simulink model "volo_radio_controller"  (Simulink 8.0)
settings: Solver=ode45  SolverMode=SingleTasking  StartTime=0.0  StopTime=1000  RelTol=1e-3
InitFcn:
  | volo_radio_controller_init
values from neighbouring files (symbols this model uses):
  cFI = fi(cMult, 1, 13, 11)    [volo_radio_controller_init.m]
  gFI = fi(gain, 1, 13, 11)    [volo_radio_controller_init.m]
  sFI = fi(sMult, 1, 13, 11)    [volo_radio_controller_init.m]
undefined symbols (not defined in the file or in its folder): gcbh, xlBlockLoadCallback, xlGetNormalizedPeriod, xlipgetpartsetting
libraries: xbsIndex_r4 x380, xbsEDKLib_r4 x1
(part 3 of 5)

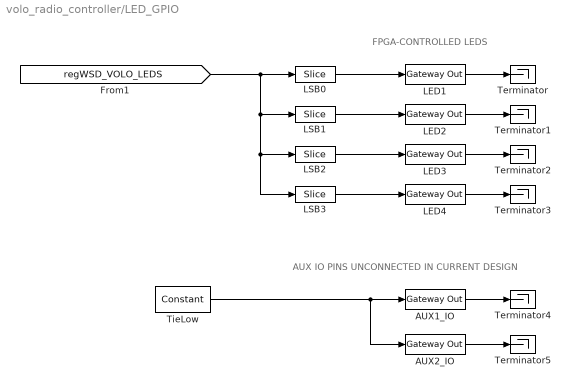
== system volo_radio_controller/LED_GPIO ==
  note: FPGA-CONTROLLED LEDS
  note: AUX IO PINS UNCONNECTED IN CURRENT DESIGN
  AUX1_IO : xbsIndex_r4/Gateway Out  inherit_from_input=off  hdl_port=off  timing_constraint=None  locs_specified=off  LOCs={}  UseAsDAC=off  DACChannel='1'  block_type=gatewayout
      settings: xl_area=[0 0 0 0 1 0 0]
  AUX2_IO : xbsIndex_r4/Gateway Out  inherit_from_input=off  hdl_port=off  timing_constraint=None  locs_specified=off  LOCs={}  UseAsDAC=off  DACChannel='1'  block_type=gatewayout
      settings: xl_area=[0 0 0 0 1 0 0]
  LED{1..4} (4 alike) : xbsIndex_r4/Gateway Out  inherit_from_input=off  hdl_port=on  timing_constraint=None  locs_specified=off  LOCs={}  UseAsDAC=off  DACChannel='1'  block_type=gatewayout
      settings: infoedit="Gateway out block.  Converts Xilinx fixed-point or floating-point type inputs into ouputs of type Simulink integer, single, double, or fixed point.<br><br>Hardware notes:  In hardware these blocks become top level output ports or are discarded, depending on how they are configured."  xl_area=[0 0 0 0 1 0 0]
  LSB0 : xbsIndex_r4/Slice  nbits=1  boolean_output=off  mode=Lower Bit Location + Width  bit1=0  base1=MSB of Input  bit0=0  base0=LSB of Input  dbl_ovrd=off  block_type=slice
      settings: block_version=8.2
  LSB1 : xbsIndex_r4/Slice  nbits=1  boolean_output=off  mode=Lower Bit Location + Width  bit1=0  base1=MSB of Input  bit0=1  base0=LSB of Input  dbl_ovrd=off  block_type=slice
      settings: block_version=8.2
  LSB2 : xbsIndex_r4/Slice  nbits=1  boolean_output=off  mode=Lower Bit Location + Width  bit1=0  base1=MSB of Input  bit0=2  base0=LSB of Input  dbl_ovrd=off  block_type=slice
      settings: block_version=8.2
  LSB3 : xbsIndex_r4/Slice  nbits=1  boolean_output=off  mode=Lower Bit Location + Width  bit1=0  base1=MSB of Input  bit0=3  base0=LSB of Input  dbl_ovrd=off  block_type=slice
      settings: block_version=8.2
  Terminator{,1..5} (6 alike) : Terminator
  TieLow : xbsIndex_r4/Constant  const=0  gui_display_data_type=Fixed-point  arith_type=Unsigned  n_bits=1  bin_pt=0  preci_type=Single  exp_width=8  frac_width=24  explicit_period=off  period=1  equ=P=C  opselect=C  inp2=PCIN>>17  opr=+  inp1=P  carry=CIN  dbl_ovrd=off  block_type=constant
  wires:
  LED1/1 -> Terminator/1
  LED2/1 -> Terminator1/1
  LED3/1 -> Terminator2/1
  LED4/1 -> Terminator3/1
  AUX1_IO/1 -> Terminator4/1
  AUX2_IO/1 -> Terminator5/1
  LSB0/1 -> LED1/1
  LSB1/1 -> LED2/1
  LSB2/1 -> LED3/1
  LSB3/1 -> LED4/1
  [regWSD_VOLO_LEDS] -> LSB0/1, LSB1/1, LSB2/1, LSB3/1
  TieLow/1 -> AUX1_IO/1, AUX2_IO/1

== system volo_radio_controller/Older Revision Notes ==
  note: Ryan - August 05, 2013
      | -------------------------------------
      | Naren - August 13, 2013 - 4.00.d
      | ** Added FP multiplies to IQ Calibration **
      | -----------------------------------
      | Ryan - August 21, 2013 - 4.00.e
      | Replaced Tx/Rx switching delay with single
      | one-shot rather than multiple delay lines:
      | regWSD_TxRxSwitchingDelayCount
      | -----------------------------------
      | 4.00.f - August 24 - Added internal UART out lines
      | with a sane naming convention such that it's easy:
      | internat TX to internal TX, external TX to external TX REG
      | -----------------------------------
      | 4.00.g - Sept 25, 2013 - Modified TXMUX to replace match-filtered
      | Rx loopback with constant-zero signals. This should help
      | with automatic calibration. REG
      | -----------------------------------
      | 4.00.h - Oct 1, 2013 - Added "ISSWAPPED" option to DDS in order
      | to programmatically mirror the SSB exponential across DC. This lets
      | us match the calibration proceedure Lime provided exactly. REG.
      | -----------------------------------
      | 4.00.j - Oct 2, 2013 - Added "ALIGNTESTACTIVE" option to DDS so
      | we can test the I/Q phase alignment. This is a test mode ONLY. REG.
      | -----------------------------------
      | 4.00.k - Oct 13, 2013 - Added "WSD_RXSWITCHINGDELAYCOUNT",
      | "WSD_SPIWAITDELAYCOUNT," and "regWSD_En_ForceSPILow" registers
      | and enable bits in order to control new Tx/Rx delay blocks in the radio controller.
      | The idea behind these is to provide the switching delays required by the SPI,
      | but in a configurable manner. Also delegate between AGC and Tx/Rx swtiching control
      | of the LMS SPI bus. This will be tricky.
      | -----------------------------------

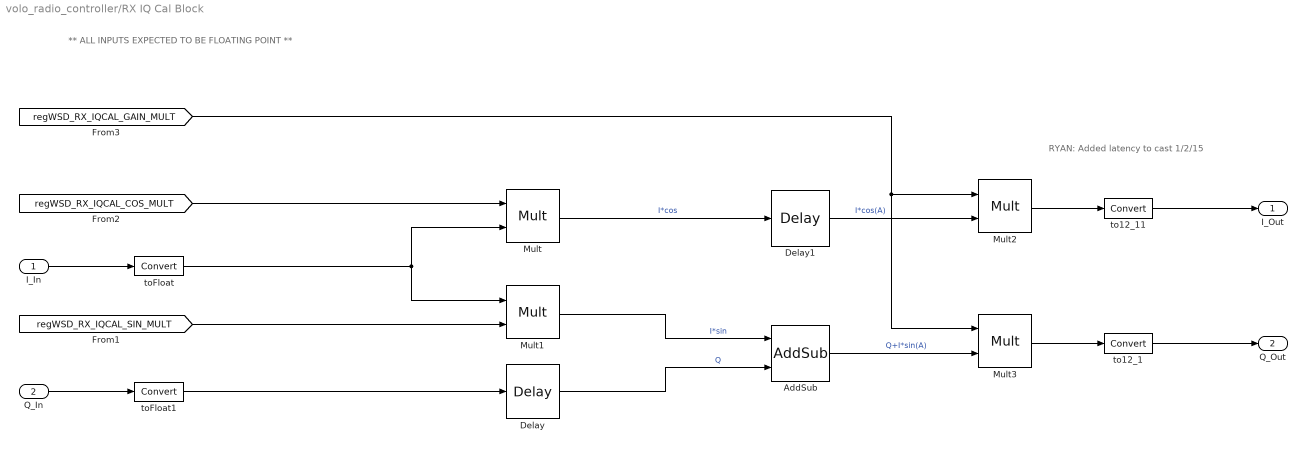
== system volo_radio_controller/RX IQ Cal Block ==
  note: RYAN: Added latency to cast 1/2/15
  note: ** ALL INPUTS EXPECTED TO BE FLOATING POINT **
  I_In : Inport
  Q_In : Inport  Port=2
  AddSub : xbsIndex_r4/AddSub  mode=Addition  use_carryin=off  use_carryout=off  en=off  latency=1  precision=Full  arith_type="Signed  (2's comp)"  n_bits=13  bin_pt=11  quantization="Round  (unbiased: +/- Inf)"  overflow=Flag as error  dbl_ovrd=off  use_behavioral_HDL=off  hw_selection=Fabric  pipelined=off  block_type=addsub
  Delay : xbsIndex_r4/Delay  rst=off  infoeditControl=Selection of Reset will increase slice count due to use of real FFs and instead of SRLs  en=off  latency=3  dbl_ovrd=off  reg_retiming=off  block_type=delay
  Delay1 : xbsIndex_r4/Delay  rst=off  infoeditControl=Selection of Reset will increase slice count due to use of real FFs and instead of SRLs  en=off  latency=1  dbl_ovrd=off  reg_retiming=off  block_type=delay
  Mult : xbsIndex_r4/Mult  precision=Full  arith_type="Signed  (2's comp)"  n_bits=13  bin_pt=11  quantization="Round  (unbiased: +/- Inf)"  overflow=Saturate  en=off  latency=3  dbl_ovrd=off  use_behavioral_HDL=off  opt=Speed  use_embedded=on  optimum_pipeline=off  pipeline=on  use_rpm=on  placement_style=Triangular  block_type=mult
  Mult1 : xbsIndex_r4/Mult  precision=Full  arith_type="Signed  (2's comp)"  n_bits=13  bin_pt=11  quantization="Round  (unbiased: +/- Inf)"  overflow=Saturate  en=off  latency=3  dbl_ovrd=off  use_behavioral_HDL=off  opt=Speed  use_embedded=on  optimum_pipeline=off  pipeline=on  use_rpm=on  placement_style=Triangular  block_type=mult
  Mult2 : xbsIndex_r4/Mult  precision=Full  arith_type="Signed  (2's comp)"  n_bits=12  bin_pt=11  quantization="Round  (unbiased: +/- Inf)"  overflow=Flag as error  en=off  latency=3  dbl_ovrd=off  use_behavioral_HDL=off  opt=Speed  use_embedded=on  optimum_pipeline=off  pipeline=on  use_rpm=on  placement_style=Triangular  block_type=mult
  Mult3 : xbsIndex_r4/Mult  precision=Full  arith_type="Signed  (2's comp)"  n_bits=12  bin_pt=11  quantization="Round  (unbiased: +/- Inf)"  overflow=Saturate  en=off  latency=3  dbl_ovrd=off  use_behavioral_HDL=off  opt=Speed  use_embedded=on  optimum_pipeline=off  pipeline=on  use_rpm=on  placement_style=Triangular  block_type=mult
  to12_1 : xbsIndex_r4/Convert  gui_display_data_type=Fixed-point  arith_type="Signed  (2's comp)"  n_bits=12  bin_pt=11  float_type=Single  exp_bits=8  fraction_bits=24  quantization="Round  (unbiased: +/- Inf)"  overflow=Saturate  en=off  latency=1  dbl_ovrd=off  pipeline=off  block_type=convert
  to12_11 : xbsIndex_r4/Convert  gui_display_data_type=Fixed-point  arith_type="Signed  (2's comp)"  n_bits=12  bin_pt=11  float_type=Single  exp_bits=8  fraction_bits=24  quantization="Round  (unbiased: +/- Inf)"  overflow=Saturate  en=off  latency=1  dbl_ovrd=off  pipeline=off  block_type=convert
  toFloat : xbsIndex_r4/Convert  gui_display_data_type=Floating-point  arith_type=Floating-point  n_bits=13  bin_pt=11  float_type=Single  exp_bits=8  fraction_bits=24  quantization="Round  (unbiased: +/- Inf)"  overflow=Flag as error  en=off  latency=0  dbl_ovrd=off  pipeline=off  block_type=convert
  toFloat1 : xbsIndex_r4/Convert  gui_display_data_type=Floating-point  arith_type=Floating-point  n_bits=13  bin_pt=11  float_type=Single  exp_bits=8  fraction_bits=24  quantization="Round  (unbiased: +/- Inf)"  overflow=Flag as error  en=off  latency=0  dbl_ovrd=off  pipeline=off  block_type=convert
  I_Out : Outport
  Q_Out : Outport  Port=2
  wires:
  I_In/1 -> toFloat/1
  [regWSD_RX_IQCAL_COS_MULT] -> Mult/1
  Q_In/1 -> toFloat1/1
  Mult/1 -> Delay1/1  "I*cos"
  Mult1/1 -> AddSub/1  "I*sin"
  [regWSD_RX_IQCAL_GAIN_MULT] -> Mult3/1, Mult2/1
  Mult2/1 -> to12_11/1
  Mult3/1 -> to12_1/1
  Delay1/1 -> Mult2/2  "I*cos(A)"
  AddSub/1 -> Mult3/2  "Q+I*sin(A)"
  Delay/1 -> AddSub/2  "Q"
  [regWSD_RX_IQCAL_SIN_MULT] -> Mult1/2
  toFloat/1 -> Mult/2, Mult1/1
  toFloat1/1 -> Delay/1
  to12_11/1 -> I_Out/1
  to12_1/1 -> Q_Out/1

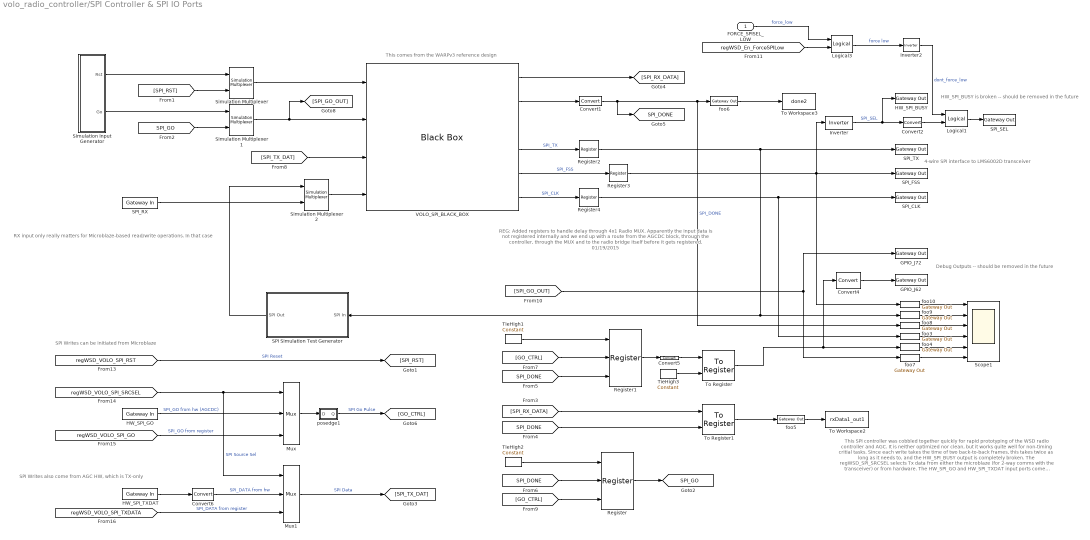
== system volo_radio_controller/SPI Controller & SPI IO Ports ==
  note: REG: Added registers to handle delay through 4x1 Radio MUX.
      | Apparently the input data is not registered internally and we end
      | up with a route from the AGCDC block, through the controller,
      | through the MUX and to the radio bridge itself before it gets
      | registered. 01/19/2015
  note: This comes from the WARPv3 reference design
  note: RX input only really matters for Microblaze-based
      | read/write operations. In that case
  note: This SPI controller was cobbled together quickly
      | for rapid prototyping of the WSD radio controller
      | and AGC. It is neither optimized nor clean, but it
      | works quite well for non-timing critial tasks. Since
      | each write takes the time of two back-to-back
      | frames, this takes twice as long as it needs to, and
      | the HW_SPI_BUSY output is completely broken.
      |
      | The regWSD_SPI_SRCSEL selects Tx data from
      | either the microblaze (for 2-way comms with the
      | transceiver) or from hardware. The HW_SPI_GO
      | and HW_SPI_TXDAT input ports come directly
      | from the WSD_AGCDC block
      |
      | Created: June 2013
      | Author: Narendra Anand (nanand@rice.edu)
      | Comments: Ryan E. Guerra (me@ryaneguerra.com)
  note: SPI Writes also come
      | from AGC HW, which is TX-only
  note: SPI Writes can be initiated from Microblaze
  note: 4-wire SPI interface to
      | LMS6002D transceiver
  note: HW_SPI_BUSY is broken -- should be removed in the future
  note: Debug Outputs -- should be removed in the future
  FORCE_SPISEL_LOW : Inport
  Convert1 : xbsIndex_r4/Convert  gui_display_data_type=Boolean  arith_type=Boolean  n_bits=32  bin_pt=0  float_type=Single  exp_bits=8  fraction_bits=24  quantization=Truncate  overflow=Wrap  en=off  latency=0  dbl_ovrd=off  pipeline=off  block_type=convert
  Convert2 : xbsIndex_r4/Convert  gui_display_data_type=Boolean  arith_type=Boolean  n_bits=32  bin_pt=0  float_type=Single  exp_bits=8  fraction_bits=24  quantization=Truncate  overflow=Wrap  en=off  latency=0  dbl_ovrd=off  pipeline=off  block_type=convert
  Convert4 : xbsIndex_r4/Convert  gui_display_data_type=Boolean  arith_type=Boolean  n_bits=32  bin_pt=0  float_type=Single  exp_bits=8  fraction_bits=24  quantization=Truncate  overflow=Wrap  en=off  latency=0  dbl_ovrd=off  pipeline=off  block_type=convert
  Convert5 : xbsIndex_r4/Convert  gui_display_data_type=Fixed-point  arith_type=Unsigned  n_bits=1  bin_pt=0  float_type=Single  exp_bits=8  fraction_bits=24  quantization=Truncate  overflow=Wrap  en=off  latency=0  dbl_ovrd=off  pipeline=off  block_type=convert
  Convert6 : xbsIndex_r4/Convert  gui_display_data_type=Fixed-point  arith_type=Unsigned  n_bits=32  bin_pt=0  float_type=Single  exp_bits=8  fraction_bits=24  quantization=Truncate  overflow=Saturate  en=off  latency=0  dbl_ovrd=off  pipeline=off  block_type=convert
  GPIO_J62 : xbsIndex_r4/Gateway Out  inherit_from_input=off  hdl_port=off  timing_constraint=None  locs_specified=off  LOCs={}  UseAsDAC=off  DACChannel='1'  block_type=gatewayout
      settings: xl_area=[0 0 0 0 1 0 0]
  GPIO_J72 : xbsIndex_r4/Gateway Out  inherit_from_input=off  hdl_port=off  timing_constraint=None  locs_specified=off  LOCs={}  UseAsDAC=off  DACChannel='1'  block_type=gatewayout
      settings: xl_area=[0 0 0 0 1 0 0]
  HW_SPI_BUSY : xbsIndex_r4/Gateway Out  inherit_from_input=off  hdl_port=off  timing_constraint=None  locs_specified=off  LOCs={}  UseAsDAC=off  DACChannel='1'  block_type=gatewayout
      settings: xl_area=[0 0 0 0 1 0 0]
  HW_SPI_GO : xbsIndex_r4/Gateway In  gui_display_data_type=Boolean  arith_type=Boolean  n_bits=1  bin_pt=0  preci_type=Single  exp_width=8  frac_width=24  quantization=Truncate  overflow=Saturate  period=1  dbl_ovrd=off  timing_constraint=None  locs_specified=off  LOCs={}  UseAsADC=off  ADCChannel='1'  inherit_from_input=off  hdl_port=on  block_type=gatewayin
      settings: xl_area=[0 0 0 0 1 0 0]
  HW_SPI_TXDAT : xbsIndex_r4/Gateway In  gui_display_data_type=Fixed-point  arith_type=Unsigned  n_bits=16  bin_pt=0  preci_type=Single  exp_width=8  frac_width=24  quantization=Truncate  overflow=Saturate  period=1  dbl_ovrd=off  timing_constraint=None  locs_specified=off  LOCs={}  UseAsADC=off  ADCChannel='1'  inherit_from_input=off  hdl_port=on  block_type=gatewayin
      settings: xl_area=[0 0 0 0 1 0 0]
  Inverter : xbsIndex_r4/Inverter  en=off  latency=0  dbl_ovrd=off  block_type=inv
  Inverter2 : xbsIndex_r4/Inverter  en=off  latency=0  dbl_ovrd=off  block_type=inv
  Logical1 : xbsIndex_r4/Logical  logical_function=AND  inputs=2  en=off  latency=0  precision=Full  arith_type=Unsigned  n_bits=16  bin_pt=0  align_bp=on  dbl_ovrd=off  block_type=logical
  Logical3 : xbsIndex_r4/Logical  logical_function=AND  inputs=2  en=off  latency=0  precision=Full  arith_type=Unsigned  n_bits=16  bin_pt=0  align_bp=on  dbl_ovrd=off  block_type=logical
  Mux : xbsIndex_r4/Mux  inputs=2  en=off  latency=0  precision=Full  arith_type=Unsigned  n_bits=16  bin_pt=14  quantization=Truncate  overflow=Wrap  dbl_ovrd=off  block_type=mux
  Mux1 : xbsIndex_r4/Mux  inputs=2  en=off  latency=0  precision=Full  arith_type=Unsigned  n_bits=16  bin_pt=14  quantization=Truncate  overflow=Wrap  dbl_ovrd=off  block_type=mux
  Register : xbsIndex_r4/Register  init=0  rst=on  en=on  dbl_ovrd=off  block_type=register
  Register1 : xbsIndex_r4/Register  init=0  rst=on  en=on  dbl_ovrd=off  block_type=register
  Register2 : xbsIndex_r4/Register  init=0  rst=off  en=off  dbl_ovrd=off  block_type=register
  Register3 : xbsIndex_r4/Register  init=0  rst=off  en=off  dbl_ovrd=off  block_type=register
  Register4 : xbsIndex_r4/Register  init=0  rst=off  en=off  dbl_ovrd=off  block_type=register
  SPI Simulation Test Generator : Subsystem
  SPI_CLK : xbsIndex_r4/Gateway Out  inherit_from_input=off  hdl_port=on  timing_constraint=None  locs_specified=off  LOCs={}  UseAsDAC=off  DACChannel='1'  block_type=gatewayout
      settings: infoedit="Gateway out block.  Converts Xilinx fixed-point or floating-point type inputs into ouputs of type Simulink integer, single, double, or fixed point.<br><br>Hardware notes:  In hardware these blocks become top level output ports or are discarded, depending on how they are configured."  xl_area=[0 0 0 0 1 0 0]
  SPI_FSS : xbsIndex_r4/Gateway Out  inherit_from_input=off  hdl_port=on  timing_constraint=None  locs_specified=off  LOCs={}  UseAsDAC=off  DACChannel='1'  block_type=gatewayout
      settings: infoedit="Gateway out block.  Converts Xilinx fixed-point or floating-point type inputs into ouputs of type Simulink integer, single, double, or fixed point.<br><br>Hardware notes:  In hardware these blocks become top level output ports or are discarded, depending on how they are configured."  xl_area=[0 0 0 0 1 0 0]
  SPI_RX : xbsIndex_r4/Gateway In  gui_display_data_type=Fixed-point  arith_type=Unsigned  n_bits=1  bin_pt=0  preci_type=Single  exp_width=8  frac_width=24  quantization=Truncate  overflow=Saturate  period=1  dbl_ovrd=off  timing_constraint=None  locs_specified=off  LOCs={}  UseAsADC=off  ADCChannel='1'  inherit_from_input=off  hdl_port=on  block_type=gatewayin
      settings: xl_area=[0 0 0 0 1 0 0]
  SPI_SEL : xbsIndex_r4/Gateway Out  inherit_from_input=off  hdl_port=on  timing_constraint=None  locs_specified=off  LOCs={}  UseAsDAC=off  DACChannel='1'  block_type=gatewayout
      settings: infoedit="Gateway out block.  Converts Xilinx fixed-point or floating-point type inputs into ouputs of type Simulink integer, single, double, or fixed point.<br><br>Hardware notes:  In hardware these blocks become top level output ports or are discarded, depending on how they are configured."  xl_area=[0 0 0 0 1 0 0]
  SPI_TX : xbsIndex_r4/Gateway Out  inherit_from_input=off  hdl_port=on  timing_constraint=None  locs_specified=off  LOCs={}  UseAsDAC=off  DACChannel='1'  block_type=gatewayout
      settings: infoedit="Gateway out block.  Converts Xilinx fixed-point or floating-point type inputs into ouputs of type Simulink integer, single, double, or fixed point.<br><br>Hardware notes:  In hardware these blocks become top level output ports or are discarded, depending on how they are configured."  xl_area=[0 0 0 0 1 0 0]
  Scope1 : Scope  NumInputPorts=6
      settings: YMin=-5~-2~-5~-5~-5~-5  YMax=5~2~5~5~5~5
  Simulation Input Generator : Subsystem
  Simulation Multiplexer : xbsIndex_r4/Simulation Multiplexer  sim_sel=1  hw_sel=2  block_type=simmux
      settings: infoedit="Distinguish input subsystems as \"simulation only\" and \"generation only\".  The input specified For Simulation will be used during Simulink simulation.  The input specified For Generation will be used during code generation.  This block will typically be used on the output of a HW Co-Simulation, Black Box, or ModelSim subsystem.<br><br>Hardware Notes: This block costs nothing."
  Simulation Multiplexer1 : xbsIndex_r4/Simulation Multiplexer  sim_sel=1  hw_sel=2  block_type=simmux
      settings: infoedit="Distinguish input subsystems as \"simulation only\" and \"generation only\".  The input specified For Simulation will be used during Simulink simulation.  The input specified For Generation will be used during code generation.  This block will typically be used on the output of a HW Co-Simulation, Black Box, or ModelSim subsystem.<br><br>Hardware Notes: This block costs nothing."
  Simulation Multiplexer2 : xbsIndex_r4/Simulation Multiplexer  sim_sel=1  hw_sel=2  block_type=simmux
      settings: infoedit="Distinguish input subsystems as \"simulation only\" and \"generation only\".  The input specified For Simulation will be used during Simulink simulation.  The input specified For Generation will be used during code generation.  This block will typically be used on the output of a HW Co-Simulation, Black Box, or ModelSim subsystem.<br><br>Hardware Notes: This block costs nothing."
  TieHigh1 : xbsIndex_r4/Constant  const=1  gui_display_data_type=Boolean  arith_type=Boolean  n_bits=1  bin_pt=0  preci_type=Single  exp_width=8  frac_width=24  explicit_period=on  period=1  equ=P=C  opselect=C  inp2=PCIN>>17  opr=+  inp1=P  carry=CIN  dbl_ovrd=off  block_type=constant
  TieHigh2 : xbsIndex_r4/Constant  const=1  gui_display_data_type=Boolean  arith_type=Boolean  n_bits=1  bin_pt=0  preci_type=Single  exp_width=8  frac_width=24  explicit_period=on  period=1  equ=P=C  opselect=C  inp2=PCIN>>17  opr=+  inp1=P  carry=CIN  dbl_ovrd=off  block_type=constant
  TieHigh3 : xbsIndex_r4/Constant  const=1  gui_display_data_type=Boolean  arith_type=Boolean  n_bits=1  bin_pt=0  preci_type=Single  exp_width=8  frac_width=24  explicit_period=on  period=1  equ=P=C  opselect=C  inp2=PCIN>>17  opr=+  inp1=P  carry=CIN  dbl_ovrd=off  block_type=constant
  To Register : xbsIndex_r4/To Register  shared_memory_name='VOLO_SPI_DONE'  init=1  ownership=Locally owned and initialized  explicit_data_type=on  gui_display_data_type=Fixed-point  arith_type=Unsigned  n_bits=1  bin_pt=0  preci_type=Single  dbl_ovrd=off  block_type=toreg
      settings: AttributesFormatString=<< %<shared_memory_name> >>  infoedit="Register block that writes data to a shared memory register.  Delay of one sample period."
  To Register1 : xbsIndex_r4/To Register  shared_memory_name='VOLO_SPI_RXDAT'  init=0  ownership=Locally owned and initialized  explicit_data_type=on  gui_display_data_type=Fixed-point  arith_type=Unsigned  n_bits=32  bin_pt=0  preci_type=Single  dbl_ovrd=off  block_type=toreg
      settings: AttributesFormatString=<< %<shared_memory_name> >>  infoedit="Register block that writes data to a shared memory register.  Delay of one sample period."
  To Workspace2 : ToWorkspace  VariableName=rxData1_out1  SampleTime=-1
  To Workspace3 : ToWorkspace  VariableName=done2  SampleTime=-1
  VOLO_SPI_BLACK_BOX : xbsIndex_r4/Black Box  init_code=volo_spi_io_config  sim_method=ISE Simulator  verbose=off  block_type=blackbox2
  foo{3..10} (8 alike) : xbsIndex_r4/Gateway Out  inherit_from_input=off  hdl_port=off  timing_constraint=None  locs_specified=off  LOCs={}  UseAsDAC=off  DACChannel='1'  block_type=gatewayout
      settings: xl_area=[0 0 0 0 1 0 0]
  posedge1 : Subsystem
  tag scope: SPI_DONE=global, SPI_GO=global
  wires:
  VOLO_SPI_BLACK_BOX/6 -> Register4/1  "SPI_CLK"
  VOLO_SPI_BLACK_BOX/2 -> Convert1/1
  VOLO_SPI_BLACK_BOX/1 -> [SPI_RX_DATA]
  SPI Simulation Test Generator/1(SPI Out) -> Simulation Multiplexer2/1
  Simulation Input Generator/1(Rst) -> Simulation Multiplexer/1
  Simulation Input Generator/2(Go) -> Simulation Multiplexer1/1
  To Register/1 -> Convert4/1, foo4/1
  [SPI_RST] -> Simulation Multiplexer/2
  Simulation Multiplexer/1 -> VOLO_SPI_BLACK_BOX/1
  [regWSD_VOLO_SPI_RST] -> [SPI_RST]  "SPI Reset"
  Convert1/1 -> [SPI_DONE], foo8/1, foo6/1  "SPI_DONE"
  Convert4/1 -> GPIO_J62/1
  [SPI_GO] -> Simulation Multiplexer1/2
  Simulation Multiplexer1/1 -> [SPI_GO_OUT], VOLO_SPI_BLACK_BOX/2
  foo4/1 -> Scope1/5
  foo6/1 -> To Workspace3/1
  VOLO_SPI_BLACK_BOX/4 -> Register2/1  "SPI_TX"
  SPI_RX/1 -> Simulation Multiplexer2/2
  [SPI_TX_DAT] -> VOLO_SPI_BLACK_BOX/3
  Simulation Multiplexer2/1 -> VOLO_SPI_BLACK_BOX/4
  TieHigh2/1 -> Register/1
  Register/1 -> [SPI_GO]
  [SPI_DONE] -> Register/2
  TieHigh3/1 -> To Register/2
  Register1/1 -> Convert5/1
  TieHigh1/1 -> Register1/1
  [SPI_DONE] -> Register1/3
  Convert5/1 -> To Register/1
  [GO_CTRL] -> Register1/2
  posedge1/1(Q) -> [GO_CTRL]  "SPI Go Pulse"
  [GO_CTRL] -> Register/3
  [SPI_GO_OUT] -> GPIO_J72/1, foo7/1
  [regWSD_VOLO_SPI_GO] -> Mux/3  "SPI_GO from register"
  Mux/1 -> posedge1/1(D)
  [regWSD_VOLO_SPI_TXDATA] -> Mux1/3  "SPI_DATA from register"
  Mux1/1 -> [SPI_TX_DAT]  "SPI Data"
  HW_SPI_TXDAT/1 -> Convert6/1
  Convert6/1 -> Mux1/2  "SPI_DATA from hw"
  [regWSD_VOLO_SPI_SRCSEL] -> Mux/1, Mux1/1  "SPI Source Sel"
  Inverter/1 -> HW_SPI_BUSY/1, Convert2/1  "SPI_SEL"
  VOLO_SPI_BLACK_BOX/5 -> Register3/1  "SPI_FSS"
  foo3/1 -> Scope1/4
  [SPI_RX_DATA] -> To Register1/1
  [SPI_DONE] -> To Register1/2
  foo5/1 -> To Workspace2/1
  To Register1/1 -> foo5/1
  foo7/1 -> Scope1/6
  foo8/1 -> Scope1/3
  foo9/1 -> Scope1/2
  foo10/1 -> Scope1/1
  HW_SPI_GO/1 -> Mux/2  "SPI_GO from hw (AGCDC)"
  Logical1/1 -> SPI_SEL/1
  FORCE_SPISEL_LOW/1 -> Logical3/1  "force_low"
  Inverter2/1 -> Logical1/1  "dont_force_low"
  Convert2/1 -> Logical1/2
  Logical3/1 -> Inverter2/1  "force low"
  [regWSD_En_ForceSPILow] -> Logical3/2
  Register2/1 -> SPI Simulation Test Generator/1(SPI In), foo9/1, SPI_TX/1
  Register3/1 -> Inverter/1, SPI_FSS/1, foo10/1
  Register4/1 -> SPI_CLK/1, foo3/1

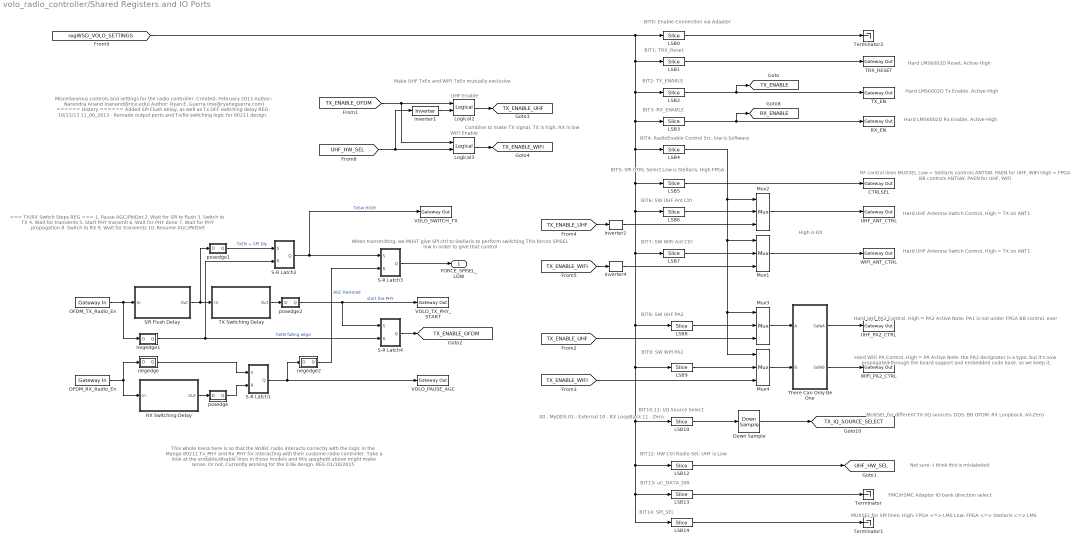
== system volo_radio_controller/Shared Registers and IO Ports ==
  note: This whole mess here is so that the WURC radio interacts correctly with
      | the logic in the Mango 80211 Tx_PHY and Rx_PHY for interacting with
      | their custome radio controller. Take a look at the endable/disable lines
      | in those models and this spaghetti above might make sense. Or not.
      | Currently working for the 0.96 design.
      | REG 01/18/2015
  note: Make UHF TxEn and WiFi TxEn mutually exclusive
  note: === TX/RX Switch Steps REG ===
      | 1. Pause AGC/PktDet
      | 2. Wait for SPI to flush
      | 3. Switch to TX
      | 4. Wait for transients
      | 5. Start PHY transmit
      | 6. Wait for PHY done
      | 7. Wait for PHY propagation
      | 8. Switch to RX
      | 9. Wait for transients
      | 10. Resume AGC/PktDet
  note: When transmitting, we MUST give SPI ctrl
      | to Stellaris to perform switching
      | This forces SPISEL low in order to give
      | that control
  note: Miscellaneous controls and settings for the radio controller.
      |
      | Created: February 2013
      | Author: Narendra Anand (nanand@rice.edu)
      | Author: Ryan E. Guerra (me@ryaneguerra.com)
      |
      | ====== History ======
      | Added SPI Flush delay, as well as Tx OFF switching delay REG 10/13/13
      | 11_06_2013 - Remade output ports and Tx/Rx switching logic for 80211 design.
  note: MUXSEL for SPI lines:
      | High: FPGA <=> LMS
      | Low: FPGA <=> Stellaris <=> LMS
  note: FMC/HSMC Adaptor
      | IO bank direction select
  note: Not sure--I think this is mislabeled
  note: MUXSEL for different TX I/Q sources:
      | DDS, BB OFDM, RX Loopback, All-Zero
  note: Hard UHF PA2 Control, High = PA2 Active
      | Note: PA1 is not under FPGA BB control, ever
  note: RF control lines MUXSEL
      | Low = Stellaris controls ANTSW, PAEN for UHF, WIFI
      | High = FPGA BB controls ANTSW, PAEN for UHF, WIFI
  note: Hard WiFi PA Control, High = PA Active
      | Note: the PA2 designator is a typo, but it's
      | now propagated through the board support
      | and embedded code base, so we keep it.
  note: Hard UHF Antenna Switch Control, High = TX on ANT1
  note: Hard UHF Antenna Switch Control, High = TX on ANT1
  note: Hard LMS6002D Rx Enable, Active-High
  note: Hard LMS6002D Tx Enable, Active-High
  note: Hard LMS6002D Reset, Active-High
  note: BIT14: SPI_SEL
  note: BIT13: uC_DATA_DIR
  note: BIT10,11: I/Q Source Select
  note: UHF Enable
  note: High is RX
  note: WIFI Enable
  note: Combine to make TX signal.
      | TX is high, RX is low
  note: BIT12: HW Ctrl Radio Sel: UHF is Low
  note: BIT9: SW Wifi PA2
  note: BIT8: SW UHF PA2
  note: BIT7: SW WIFI Ant Ctrl
  note: BIT6: SW UHF Ant Ctrl
  note: BIT0: Enable Connection via Adapter
  note: BIT1: TRX_Reset
  note: BIT2: TX_ENABLE
  note: BIT3: RX_ENABLE
  note: BIT4: RadioEnable Control Src, low is Software
  note: BIT5: SPI CTRL Select
      | Low is Stellaris, High FPGA
  note: 00 - MyDDS
      | 01 - External
      | 10 - RX LoopBack
      | 11 - Zero
  CTRLSEL : xbsIndex_r4/Gateway Out  inherit_from_input=off  hdl_port=off  timing_constraint=None  locs_specified=off  LOCs={}  UseAsDAC=off  DACChannel='1'  block_type=gatewayout
      settings: xl_area=[0 0 0 0 1 0 0]
  Down Sample : xbsIndex_r4/Down Sample  sample_ratio=2  sample_phase="Last Value of Frame  (most efficient)"  en=off  latency=1  dbl_ovrd=off  block_type=dsamp
  Inverter1 : xbsIndex_r4/Inverter  en=off  latency=0  dbl_ovrd=off  block_type=inv
  Inverter2 : xbsIndex_r4/Inverter  en=off  latency=0  dbl_ovrd=off  block_type=inv
  Inverter4 : xbsIndex_r4/Inverter  en=off  latency=0  dbl_ovrd=off  block_type=inv
  LSB0 : xbsIndex_r4/Slice  nbits=1  boolean_output=on  mode=Lower Bit Location + Width  bit1=0  base1=MSB of Input  bit0=0  base0=LSB of Input  dbl_ovrd=off  block_type=slice
      settings: block_version=8.2
  LSB1 : xbsIndex_r4/Slice  nbits=1  boolean_output=on  mode=Lower Bit Location + Width  bit1=0  base1=MSB of Input  bit0=1  base0=LSB of Input  dbl_ovrd=off  block_type=slice
      settings: block_version=8.2
  LSB10 : xbsIndex_r4/Slice  nbits=2  boolean_output=off  mode=Lower Bit Location + Width  bit1=0  base1=MSB of Input  bit0=10  base0=LSB of Input  dbl_ovrd=off  block_type=slice
      settings: block_version=8.2
  LSB12 : xbsIndex_r4/Slice  nbits=1  boolean_output=on  mode=Lower Bit Location + Width  bit1=0  base1=MSB of Input  bit0=12  base0=LSB of Input  dbl_ovrd=off  block_type=slice
      settings: block_version=8.2
  LSB13 : xbsIndex_r4/Slice  nbits=1  boolean_output=on  mode=Lower Bit Location + Width  bit1=0  base1=MSB of Input  bit0=13  base0=LSB of Input  dbl_ovrd=off  block_type=slice
      settings: block_version=8.2
  LSB14 : xbsIndex_r4/Slice  nbits=1  boolean_output=on  mode=Lower Bit Location + Width  bit1=0  base1=MSB of Input  bit0=14  base0=LSB of Input  dbl_ovrd=off  block_type=slice
      settings: block_version=8.2
  LSB2 : xbsIndex_r4/Slice  nbits=1  boolean_output=on  mode=Lower Bit Location + Width  bit1=0  base1=MSB of Input  bit0=2  base0=LSB of Input  dbl_ovrd=off  block_type=slice
      settings: block_version=8.2
  LSB3 : xbsIndex_r4/Slice  nbits=1  boolean_output=on  mode=Lower Bit Location + Width  bit1=0  base1=MSB of Input  bit0=3  base0=LSB of Input  dbl_ovrd=off  block_type=slice
      settings: block_version=8.2
  LSB4 : xbsIndex_r4/Slice  nbits=1  boolean_output=on  mode=Lower Bit Location + Width  bit1=0  base1=MSB of Input  bit0=4  base0=LSB of Input  dbl_ovrd=off  block_type=slice
      settings: block_version=8.2
  LSB5 : xbsIndex_r4/Slice  nbits=1  boolean_output=on  mode=Lower Bit Location + Width  bit1=0  base1=MSB of Input  bit0=5  base0=LSB of Input  dbl_ovrd=off  block_type=slice
      settings: block_version=8.2
  LSB6 : xbsIndex_r4/Slice  nbits=1  boolean_output=on  mode=Lower Bit Location + Width  bit1=0  base1=MSB of Input  bit0=6  base0=LSB of Input  dbl_ovrd=off  block_type=slice
      settings: block_version=8.2
  LSB7 : xbsIndex_r4/Slice  nbits=1  boolean_output=on  mode=Lower Bit Location + Width  bit1=0  base1=MSB of Input  bit0=7  base0=LSB of Input  dbl_ovrd=off  block_type=slice
      settings: block_version=8.2
  LSB8 : xbsIndex_r4/Slice  nbits=1  boolean_output=on  mode=Lower Bit Location + Width  bit1=0  base1=MSB of Input  bit0=8  base0=LSB of Input  dbl_ovrd=off  block_type=slice
      settings: block_version=8.2
  LSB9 : xbsIndex_r4/Slice  nbits=1  boolean_output=on  mode=Lower Bit Location + Width  bit1=0  base1=MSB of Input  bit0=9  base0=LSB of Input  dbl_ovrd=off  block_type=slice
      settings: block_version=8.2
  Logical2 : xbsIndex_r4/Logical  logical_function=AND  inputs=2  en=off  latency=0  precision=Full  arith_type=Unsigned  n_bits=16  bin_pt=0  align_bp=on  dbl_ovrd=off  block_type=logical
  Logical3 : xbsIndex_r4/Logical  logical_function=AND  inputs=2  en=off  latency=0  precision=Full  arith_type=Unsigned  n_bits=16  bin_pt=0  align_bp=on  dbl_ovrd=off  block_type=logical
  Mux{1..4} (4 alike) : xbsIndex_r4/Mux  inputs=2  en=off  latency=0  precision=Full  arith_type=Unsigned  n_bits=16  bin_pt=14  quantization=Truncate  overflow=Wrap  dbl_ovrd=off  block_type=mux
  OFDM_RX_Radio_En : xbsIndex_r4/Gateway In  gui_display_data_type=Boolean  arith_type=Boolean  n_bits=12  bin_pt=11  preci_type=Single  exp_width=8  frac_width=24  quantization="Round  (unbiased: +/- Inf)"  overflow=Saturate  period=1  dbl_ovrd=off  timing_constraint=None  locs_specified=off  LOCs={}  UseAsADC=off  ADCChannel='1'  inherit_from_input=off  hdl_port=on  block_type=gatewayin
      settings: xl_area=[0 0 0 0 12 0 0]
  OFDM_TX_Radio_En : xbsIndex_r4/Gateway In  gui_display_data_type=Boolean  arith_type=Boolean  n_bits=12  bin_pt=11  preci_type=Single  exp_width=8  frac_width=24  quantization="Round  (unbiased: +/- Inf)"  overflow=Saturate  period=1  dbl_ovrd=off  timing_constraint=None  locs_specified=off  LOCs={}  UseAsADC=off  ADCChannel='1'  inherit_from_input=off  hdl_port=on  block_type=gatewayin
      settings: xl_area=[0 0 0 0 12 0 0]
  RX Switching Delay : Subsystem
  RX_EN : xbsIndex_r4/Gateway Out  inherit_from_input=off  hdl_port=on  timing_constraint=None  locs_specified=off  LOCs={}  UseAsDAC=off  DACChannel='1'  block_type=gatewayout
      settings: infoedit="Gateway out block.  Converts Xilinx fixed-point or floating-point type inputs into ouputs of type Simulink integer, single, double, or fixed point.<br><br>Hardware notes:  In hardware these blocks become top level output ports or are discarded, depending on how they are configured."  xl_area=[0 0 0 0 1 0 0]
  S-R Latch1 : Subsystem
  S-R Latch2 : Subsystem
  S-R Latch3 : Subsystem
  S-R Latch4 : Subsystem
  "SPI Flush Delay " : Subsystem
  TRX_RESET : xbsIndex_r4/Gateway Out  inherit_from_input=off  hdl_port=on  timing_constraint=None  locs_specified=off  LOCs={}  UseAsDAC=off  DACChannel='1'  block_type=gatewayout
      settings: infoedit="Gateway out block.  Converts Xilinx fixed-point or floating-point type inputs into ouputs of type Simulink integer, single, double, or fixed point.<br><br>Hardware notes:  In hardware these blocks become top level output ports or are discarded, depending on how they are configured."  xl_area=[0 0 0 0 1 0 0]
  TX Switching Delay : Subsystem
  TX_EN : xbsIndex_r4/Gateway Out  inherit_from_input=off  hdl_port=on  timing_constraint=None  locs_specified=off  LOCs={}  UseAsDAC=off  DACChannel='1'  block_type=gatewayout
      settings: infoedit="Gateway out block.  Converts Xilinx fixed-point or floating-point type inputs into ouputs of type Simulink integer, single, double, or fixed point.<br><br>Hardware notes:  In hardware these blocks become top level output ports or are discarded, depending on how they are configured."  xl_area=[0 0 0 0 1 0 0]
  Terminator : Terminator
  Terminator1 : Terminator
  Terminator2 : Terminator
  There Can Only Be One : Subsystem
  UHF_ANT_CTRL : xbsIndex_r4/Gateway Out  inherit_from_input=off  hdl_port=off  timing_constraint=None  locs_specified=off  LOCs={}  UseAsDAC=off  DACChannel='1'  block_type=gatewayout
      settings: xl_area=[0 0 0 0 1 0 0]
  UHF_PA2_CTRL : xbsIndex_r4/Gateway Out  inherit_from_input=off  hdl_port=off  timing_constraint=None  locs_specified=off  LOCs={}  UseAsDAC=off  DACChannel='1'  block_type=gatewayout
      settings: xl_area=[0 0 0 0 1 0 0]
  VOLO_PAUSE_AGC : xbsIndex_r4/Gateway Out  inherit_from_input=off  hdl_port=on  timing_constraint=None  locs_specified=off  LOCs={}  UseAsDAC=off  DACChannel='1'  block_type=gatewayout
      settings: infoedit="Gateway out block.  Converts Xilinx fixed-point or floating-point type inputs into ouputs of type Simulink integer, single, double, or fixed point.<br><br>Hardware notes:  In hardware these blocks become top level output ports or are discarded, depending on how they are configured."  xl_area=[0 0 0 0 1 0 0]
  VOLO_SWITCH_TX : xbsIndex_r4/Gateway Out  inherit_from_input=off  hdl_port=on  timing_constraint=None  locs_specified=off  LOCs={}  UseAsDAC=off  DACChannel='1'  block_type=gatewayout
      settings: infoedit="Gateway out block.  Converts Xilinx fixed-point or floating-point type inputs into ouputs of type Simulink integer, single, double, or fixed point.<br><br>Hardware notes:  In hardware these blocks become top level output ports or are discarded, depending on how they are configured."  xl_area=[0 0 0 0 1 0 0]
  VOLO_TX_PHY_START : xbsIndex_r4/Gateway Out  inherit_from_input=off  hdl_port=on  timing_constraint=None  locs_specified=off  LOCs={}  UseAsDAC=off  DACChannel='1'  block_type=gatewayout
      settings: infoedit="Gateway out block.  Converts Xilinx fixed-point or floating-point type inputs into ouputs of type Simulink integer, single, double, or fixed point.<br><br>Hardware notes:  In hardware these blocks become top level output ports or are discarded, depending on how they are configured."  xl_area=[0 0 0 0 1 0 0]
  WIFI_ANT_CTRL : xbsIndex_r4/Gateway Out  inherit_from_input=off  hdl_port=off  timing_constraint=None  locs_specified=off  LOCs={}  UseAsDAC=off  DACChannel='1'  block_type=gatewayout
      settings: xl_area=[0 0 0 0 1 0 0]
  WIFI_PA2_CTRL : xbsIndex_r4/Gateway Out  inherit_from_input=off  hdl_port=off  timing_constraint=None  locs_specified=off  LOCs={}  UseAsDAC=off  DACChannel='1'  block_type=gatewayout
      settings: xl_area=[0 0 0 0 1 0 0]
  negedge : Subsystem
  negedge1 : Subsystem
  negedge2 : Subsystem
  posedge : Subsystem
  posedge1 : Subsystem
  posedge2 : Subsystem
  FORCE_SPISEL_LOW : Outport
  tag scope: RX_ENABLE=global, TX_ENABLE=global, TX_ENABLE_OFDM=global, TX_ENABLE_UHF=global, TX_ENABLE_WIFI=global, TX_IQ_SOURCE_SELECT=global, UHF_HW_SEL=global
  wires:
  [regWSD_VOLO_SETTINGS] -> LSB0/1, LSB1/1, LSB14/1, LSB13/1, LSB12/1, LSB10/1, LSB9/1, LSB8/1, LSB7/1, LSB6/1, LSB5/1, LSB4/1, LSB3/1, LSB2/1
  LSB0/1 -> Terminator2/1
  LSB1/1 -> TRX_RESET/1
  LSB2/1 -> [TX_ENABLE], TX_EN/1
  LSB3/1 -> RX_EN/1, [RX_ENABLE]
  LSB5/1 -> CTRLSEL/1
  LSB10/1 -> Down Sample/1
  Mux2/1 -> UHF_ANT_CTRL/1
  Mux1/1 -> WIFI_ANT_CTRL/1
  LSB4/1 -> Mux2/1, Mux1/1, Mux4/1, Mux3/1
  LSB6/1 -> Mux2/2
  LSB7/1 -> Mux1/2
  There Can Only Be One/1(SafeA) -> UHF_PA2_CTRL/1
  There Can Only Be One/2(SafeB) -> WIFI_PA2_CTRL/1
  LSB8/1 -> Mux3/2
  LSB9/1 -> Mux4/2
  Mux3/1 -> There Can Only Be One/1(A)
  Mux4/1 -> There Can Only Be One/2(B)
  LSB12/1 -> [UHF_HW_SEL]
  [TX_ENABLE_OFDM] -> Logical3/1, Logical2/1
  [UHF_HW_SEL] -> Inverter1/1, Logical3/2
  Inverter1/1 -> Logical2/2
  Logical3/1 -> [TX_ENABLE_WIFI]
  Logical2/1 -> [TX_ENABLE_UHF]
  [TX_ENABLE_UHF] -> Mux3/3
  [TX_ENABLE_WIFI] -> Mux4/3
  [TX_ENABLE_WIFI] -> Inverter4/1
  [TX_ENABLE_UHF] -> Inverter2/1
  Inverter2/1 -> Mux2/3
  Inverter4/1 -> Mux1/3
  LSB13/1 -> Terminator/1
  LSB14/1 -> Terminator1/1
  Down Sample/1 -> [TX_IQ_SOURCE_SELECT]
  TX Switching Delay/1(Out) -> posedge2/1(D)
  OFDM_TX_Radio_En/1 -> negedge1/1(D), "SPI Flush Delay "/1(In)
  "SPI Flush Delay "/1(Out) -> TX Switching Delay/1(In), posedge1/1(D)
  S-R Latch3/1(Q) -> FORCE_SPISEL_LOW/1
  S-R Latch2/1(Q) -> S-R Latch3/1(S), VOLO_SWITCH_TX/1  "TxSw HIGH"
  negedge/1(Q) -> S-R Latch1/1(S)
  S-R Latch1/1(Q) -> negedge2/1(D), VOLO_PAUSE_AGC/1
  OFDM_RX_Radio_En/1 -> RX Switching Delay/1(In), negedge/1(D)
  RX Switching Delay/1(Out) -> posedge/1(D)
  posedge/1(Q) -> S-R Latch1/2(R)
  S-R Latch4/1(Q) -> [TX_ENABLE_OFDM]
  posedge2/1(Q) -> S-R Latch4/1(S), VOLO_TX_PHY_START/1  "start the PHY"
  negedge1/1(Q) -> S-R Latch2/2(R), S-R Latch4/2(R)  "TxEN falling edge"
  negedge2/1(Q) -> S-R Latch3/2(R)  "AGC Restored"
  posedge1/1(Q) -> S-R Latch2/1(S)  "TxEN + SPI Dly"
